simulink model "cllc_control"  (R2022a)
settings: Solver=FixedStepDiscrete  StartTime=0.0  StopTime=Inf  FixedStep=stepsize  RelTol=1e-9  AbsTol=1e-9  EnableMultiTasking=on
model workspace (MAT data in the model file):
  A_d = [1  1  1  1  1  1  1  1  1; 2  2  2  2  2  2  2  2  2]
  dcdc_direction = 1
  iout_ref = Simulink.Parameter
  iout_ref.DataType = 'auto'
  iout_ref.Complexity = 'real'
  iout_ref.Dimensions = [0 0]
  llc1_pri_idc = Simulink.Signal
  llc1_pri_idc.DataType = 'uint16'
  llc1_pri_idc.Dimensions = -1
  llc1_pri_idc.DimensionsMode = 'Fixed'
  llc1_pri_idc.Complexity = 'real'
  llc1_pri_idc.SampleTime = -1
  llc1_pri_idc.SamplingMode = 'auto'
  llc1_pri_idc.InitialValue = '0'
  llc1_sec_idc = Simulink.Signal
  llc1_sec_idc.DataType = 'uint16'
  llc1_sec_idc.Dimensions = -1
  llc1_sec_idc.DimensionsMode = 'Fixed'
  llc1_sec_idc.Complexity = 'real'
  llc1_sec_idc.SampleTime = -1
  llc1_sec_idc.SamplingMode = 'auto'
  llc1_sec_idc.InitialValue = '0'
  ref_iout = Simulink.Signal
  ref_iout.DataType = 'uint16'
  ref_iout.Dimensions = -1
  ref_iout.DimensionsMode = 'Fixed'
  ref_iout.Complexity = 'real'
  ref_iout.SampleTime = -1
  ref_iout.SamplingMode = 'auto'
  ref_iout.InitialValue = '0'
  ref_iout_calib = Simulink.Signal
  ref_iout_calib.DataType = 'uint16'
  ref_iout_calib.Dimensions = -1
  ref_iout_calib.DimensionsMode = 'Fixed'
  ref_iout_calib.Complexity = 'real'
  ref_iout_calib.SampleTime = -1
  ref_iout_calib.SamplingMode = 'auto'
  ref_iout_calib.InitialValue = '0'
  ref_ss_llc1 = Simulink.Signal
  ref_ss_llc1.DataType = 'uint16'
  ref_ss_llc1.Dimensions = -1
  ref_ss_llc1.DimensionsMode = 'Fixed'
  ref_ss_llc1.Complexity = 'real'
  ref_ss_llc1.SampleTime = -1
  ref_ss_llc1.SamplingMode = 'auto'
  ref_ss_llc1.InitialValue = '0'
  ref_vbat = Simulink.Signal
  ref_vbat.DataType = 'uint16'
  ref_vbat.Dimensions = -1
  ref_vbat.DimensionsMode = 'Fixed'
  ref_vbat.Complexity = 'real'
  ref_vbat.SampleTime = -1
  ref_vbat.SamplingMode = 'auto'
  ref_vbat.InitialValue = '0'
  ref_vbat_calib = Simulink.Signal
  ref_vbat_calib.DataType = 'uint16'
  ref_vbat_calib.Dimensions = -1
  ref_vbat_calib.DimensionsMode = 'Fixed'
  ref_vbat_calib.Complexity = 'real'
  ref_vbat_calib.SampleTime = -1
  ref_vbat_calib.SamplingMode = 'auto'
  ref_vbat_calib.InitialValue = '0'
  vbat = Simulink.Signal
  vbat.DataType = 'uint16'
  vbat.Dimensions = -1
  vbat.DimensionsMode = 'Fixed'
  vbat.Complexity = 'real'
  vbat.SampleTime = -1
  vbat.SamplingMode = 'auto'
  vbat.InitialValue = '0'
  vbat_ref = Simulink.Parameter
  vbat_ref.DataType = 'auto'
  vbat_ref.Complexity = 'real'
  vbat_ref.Dimensions = [0 0]
  vout = Simulink.Signal
  vout.DataType = 'uint16'
  vout.Dimensions = -1
  vout.DimensionsMode = 'Fixed'
  vout.Complexity = 'real'
  vout.SampleTime = -1
  vout.SamplingMode = 'auto'
  vout.InitialValue = '0'
values from neighbouring files (symbols this model uses):
  epwmclk = 100000000.0    [cllc_data_lib.sldd]
  stepsize = 2.0E-7    [cllc_data_lib.sldd]
  var_dir_v2g = 0.0    [cllc_data_lib.sldd]
undefined symbols (not defined in the file or in its folder): f32Iout, f32VoutTarget
libraries: spsSampleandHoldLib x16, simulink_extras x6
(part 1 of 2)
settings Model: DataDictionary=cllc_data_lib.sldd  EnableAccessToBaseWorkspace=off  ExtModeTrigDuration=8  Creator=johncanas  LastModifiedBy=sgcesuser2
settings SolverCC: MaxConsecutiveMinStep=10  ZeroCrossAlgorithm=Adaptive  AlgebraicLoopSolver=TrustRegion  AutoInsertRateTranBlk=on  InsertRTBMode=Always
settings DataIOCC: SaveState=on  SignalLoggingName=SIL_signals
settings OptimizationCC: DefaultUnderspecifiedDataType=single  EnhancedBackFolding=on  PassReuseOutputArgsAs=Individual arguments  MaxStackSize=1024  OptimizeBlockOrder=speed  DifferentSizesBufferReuse=on  OptimizationCustomize=off  DenormalBehavior=FlushToZero  EfficientTunableParamExpr=on
settings DebuggingCC: IgnoredZcDiagnostic=none  MultiTaskDSMMsg=none  ParameterTunabilityLossMsg=error  UnconnectedInputMsg=warning  UnconnectedOutputMsg=warning  UnconnectedLineMsg=warning  BusObjectLabelMismatch=error  SFMachineParentedDataDiag=warning  UnderSpecifiedDimensionMsg=warning
settings HardwareCC: ProdBitPerChar=16  ProdBitPerInt=16  ProdBitPerPointer=32  ProdBitPerSizeT=32  ProdBitPerPtrDiffT=32  ProdLargestAtomicInteger=Integer  ProdLargestAtomicFloat=None  ProdWordSize=16  ProdLongLongMode=on  ProdHWDeviceType=Texas Instruments->C2000
settings ModelReferenceCC: EnableRefExpFcnMdlSchedulingChecks=off
settings SFSimCC: MATLABDynamicMemAlloc=off  CustomCodeUndefinedFunction=UseInterfaceOnly
settings RTWCC: SystemTargetFile=ert.tlc  HardwareBoard=TI Piccolo F2807x  TemplateMakefile=ert_default_tmf  GenerateReport=on  Toolchain=Texas Instruments Code Composer Studio (C2000)  IncludeHyperlinkInReport=on  LaunchReport=on  PortableWordSizes=on  GenerateTraceInfo=on  GenerateTraceReport=on  GenerateTraceReportSl=on  GenerateTraceReportSf=on  GenerateTraceReportEml=on  DLArmComputeVersion=19.05
settings CodeAppCC: ForceParamTrailComments=on  IgnoreCustomStorageClasses=off  OperatorAnnotations=on  SimulinkDataObjDesc=on  SFDataObjDesc=on  InsertBlockDesc=on
settings ERTTargetCC: CodeReplacementLibrary=TI C28x  SupportContinuousTime=on  SupportNonInlinedSFcns=on  ExtModeStaticAllocSize=2000

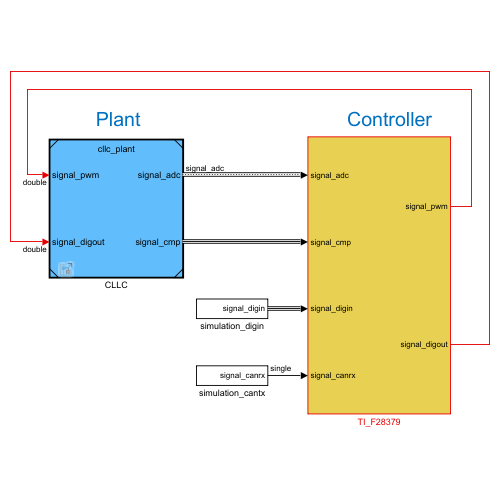
[thumbnail: Simulink's stored preview of the top-level diagram]
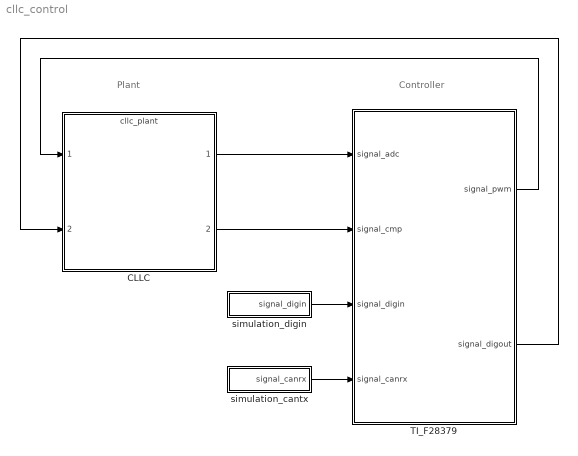
== system cllc_control ==
  note: Controller
  note: Plant
  CLLC : ModelReference  ModelNameDialog=cllc_plant.slx  SimulationMode=Normal  ModelReferenceVersion=2.76
  TI_F28379 : Subsystem
  simulation_cantx : Subsystem
  simulation_digin : Subsystem
  wires:
  CLLC/1 -> TI_F28379/1(signal_adc)
  TI_F28379/1(signal_pwm) -> CLLC/1
  TI_F28379/2(signal_digout) -> CLLC/2
  CLLC/2 -> TI_F28379/2(signal_cmp)
  simulation_digin/1(signal_digin) -> TI_F28379/3(signal_digin)
  simulation_cantx/1(signal_canrx) -> TI_F28379/4(signal_canrx)

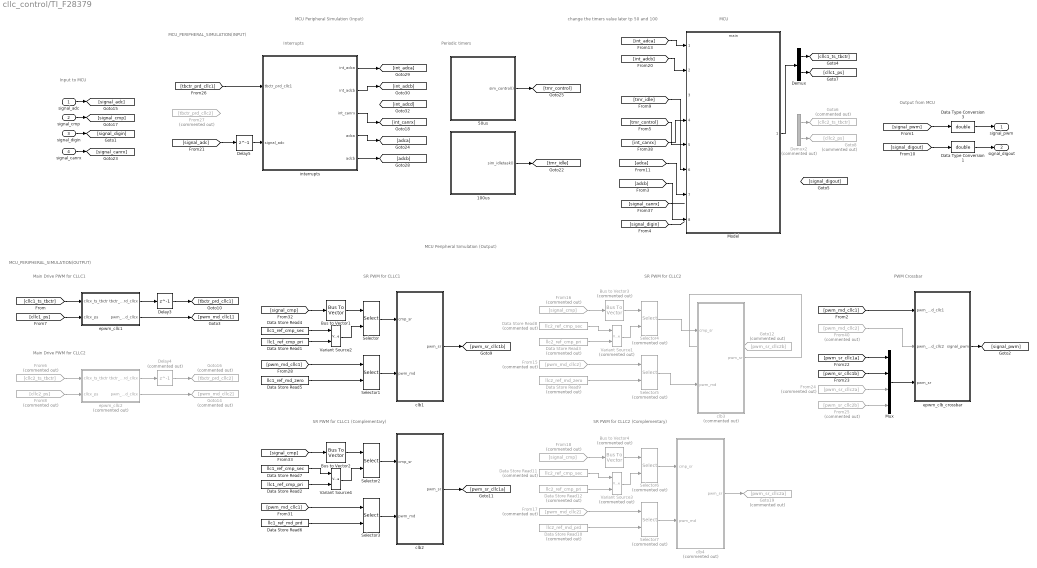
== system cllc_control/TI_F28379 ==
  note: change the timers value later tp 50 and 100
  note: MCU_PERIPHERAL_SIMULATION(OUTPUT)
  note: MCU_PERIPHERAL_SIMULATION(INPUT)
  note: MCU
  note: Input to MCU
  note: Output from MCU
  note: Interrupts
  note: Periodic timers
  note: SR PWM for CLLC2 (Complementary)
  note: SR PWM for CLLC2
  note: Main Drive PWM for CLLC2
  note: SR PWM for CLLC1 (Complementary)
  note: SR PWM for CLLC1
  note: Main Drive PWM for CLLC1
  note: PWM Crossbar
  note: MCU Peripheral Simulation (Input)
  note: MCU Peripheral Simulation (Output)
  signal_adc : Inport
  signal_cmp : Inport  Port=2
  signal_digin : Inport  Port=3
  signal_canrx : Inport  Port=4
  100us : Stateflow chart  TreatAsAtomicUnit=on  SystemSampleTime=2e-6
  50us : Stateflow chart  TreatAsAtomicUnit=on  SystemSampleTime=50e-6
  Bus to Vector1 : BusToVector
  Bus to Vector2 : BusToVector
  Bus to Vector3 : BusToVector  Commented=on
  Bus to Vector4 : BusToVector  Commented=on
  Data Store Read1 : DataStoreRead  DataStoreName=llc1_ref_cmp_pri  IndexOptions=Index vector (dialog)  Indices=1  OutputSizes=1
  Data Store Read10 : DataStoreRead  Commented=on  DataStoreName=llc2_ref_md_prd  IndexOptions=Index vector (dialog)  Indices=1  OutputSizes=1
  Data Store Read11 : DataStoreRead  Commented=on  DataStoreName=llc2_ref_cmp_sec  IndexOptions=Index vector (dialog)  Indices=1  OutputSizes=1
  Data Store Read12 : DataStoreRead  Commented=on  DataStoreName=llc2_ref_cmp_pri  IndexOptions=Index vector (dialog)  Indices=1  OutputSizes=1
  Data Store Read2 : DataStoreRead  DataStoreName=llc1_ref_cmp_pri  IndexOptions=Index vector (dialog)  Indices=1  OutputSizes=1
  Data Store Read3 : DataStoreRead  Commented=on  DataStoreName=llc2_ref_cmp_pri  IndexOptions=Index vector (dialog)  Indices=1  OutputSizes=1
  Data Store Read4 : DataStoreRead  DataStoreName=llc1_ref_cmp_sec  IndexOptions=Index vector (dialog)  Indices=1  OutputSizes=1
  Data Store Read5 : DataStoreRead  DataStoreName=llc1_ref_md_zero  IndexOptions=Index vector (dialog)  Indices=1  OutputSizes=1
  Data Store Read6 : DataStoreRead  DataStoreName=llc1_ref_md_prd  IndexOptions=Index vector (dialog)  Indices=1  OutputSizes=1
  Data Store Read7 : DataStoreRead  DataStoreName=llc1_ref_cmp_sec  IndexOptions=Index vector (dialog)  Indices=1  OutputSizes=1
  Data Store Read8 : DataStoreRead  Commented=on  DataStoreName=llc2_ref_cmp_sec  IndexOptions=Index vector (dialog)  Indices=1  OutputSizes=1
  Data Store Read9 : DataStoreRead  Commented=on  DataStoreName=llc2_ref_md_zero  IndexOptions=Index vector (dialog)  Indices=1  OutputSizes=1
  Data Type Conversion1 : DataTypeConversion  OutDataTypeStr=double  SaturateOnIntegerOverflow=off  RndMeth=Floor
  Data Type Conversion3 : DataTypeConversion  OutDataTypeStr=double  SaturateOnIntegerOverflow=off  RndMeth=Floor
  Delay3 : Delay  DelayLength=1
  Delay4 : Delay  Commented=on  DelayLength=1
  Delay5 : Delay  DelayLength=1
  Demux : Demux  Outputs=2
  Demux2 : Demux  Commented=on  Outputs=2
  From15 : From  Commented=on  GotoTag=pwm_md_cllc2
  From16 : From  Commented=on  GotoTag=signal_cmp
  From17 : From  Commented=on  GotoTag=pwm_md_cllc2
  From18 : From  Commented=on  GotoTag=signal_cmp
  From24 : From  Commented=on  GotoTag=pwm_sr_cllc2a
  From25 : From  Commented=on  GotoTag=pwm_sr_cllc2b
  From27 : From  Commented=on  GotoTag=tbctr_prd_cllc2
  From40 : From  Commented=on  GotoTag=pwm_md_cllc2
  From6 : From  Commented=on  GotoTag=cllc2_ts_tbctr
  From8 : From  Commented=on  GotoTag=cllc2_ps
  Goto12 : Goto  Commented=on  GotoTag=pwm_sr_cllc2b
  Goto14 : Goto  Commented=on  GotoTag=pwm_md_cllc2
  Goto16 : Goto  Commented=on  GotoTag=tbctr_prd_cllc2
  Goto19 : Goto  Commented=on  GotoTag=pwm_sr_cllc2a
  Goto6 : Goto  Commented=on  GotoTag=cllc2_ts_tbctr
  Goto8 : Goto  Commented=on  GotoTag=cllc2_ps
  Model : ModelReference  ModelNameDialog=main.slx  SimulationMode=Normal  ScheduleRates=on  ModelReferenceVersion=5.515
  Mux : Mux
  Selector : Selector  InputPortWidth=4  IndexOptions=Index vector (port)  Indices=[1 3]  OutputSizes=1
  Selector1 : Selector  InputPortWidth=8  IndexOptions=Index vector (port)  Indices=[1 3]  OutputSizes=1
  Selector2 : Selector  InputPortWidth=4  IndexOptions=Index vector (port)  Indices=[1 3]  OutputSizes=1
  Selector3 : Selector  InputPortWidth=8  IndexOptions=Index vector (port)  Indices=[1 3]  OutputSizes=1
  Selector4 : Selector  Commented=on  InputPortWidth=4  IndexOptions=Index vector (port)  Indices=[1 3]  OutputSizes=1
  Selector5 : Selector  Commented=on  InputPortWidth=8  IndexOptions=Index vector (port)  Indices=[1 3]  OutputSizes=1
  Selector6 : Selector  Commented=on  InputPortWidth=4  IndexOptions=Index vector (port)  Indices=[1 3]  OutputSizes=1
  Selector7 : Selector  Commented=on  InputPortWidth=8  IndexOptions=Index vector (port)  Indices=[1 3]  OutputSizes=1
  Variant Source1 : VariantSource  Commented=on
      settings: AllowZeroVariantControls=on
  Variant Source2 : VariantSource
      settings: AllowZeroVariantControls=on
  Variant Source3 : VariantSource  Commented=on
      settings: AllowZeroVariantControls=on
  Variant Source4 : VariantSource
      settings: AllowZeroVariantControls=on
  clb1 : Subsystem
  clb2 : Subsystem
  clb3 : Subsystem  Commented=on
  clb4 : Subsystem  Commented=on
  epwm_clb_crossbar : Subsystem
  epwm_cllc1 : Subsystem
  epwm_cllc2 : Subsystem  Commented=on
  interrupts : Subsystem
  signal_pwm : Outport  VectorParamsAs1DForOutWhenUnconnected=off
  signal_digout : Outport  Port=2
  wires:
  Model/1 -> Demux/1
  Demux/1 -> [cllc1_ts_tbctr]
  Demux/2 -> [cllc1_ps]
  [signal_digout] -> Data Type Conversion1/1
  Demux2/2 -> Goto8/1
  Demux2/1 -> Goto6/1
  signal_cmp/1 -> [signal_cmp]
  ? -> [signal_digout]
  signal_adc/1 -> [signal_adc]
  [int_adca] -> Model/1
  [int_adcb] -> Model/2
  ? -> Model/3
  signal_digin/1 -> [signal_digin]
  signal_canrx/1 -> [signal_canrx]
  [signal_digin] -> ?
  [signal_canrx] -> ?
  ? -> [int_adcd]
  interrupts/5(adcb) -> [adcb]
  interrupts/4(adca) -> [adca]
  Delay5/1 -> interrupts/2(signal_adc)
  [tbctr_prd_cllc1] -> interrupts/1(tbctr_prd_cllc1)
  interrupts/3(int_canrx) -> [int_canrx]
  interrupts/1(int_adca) -> [int_adca]
  50us/1(sim_control()) -> [tmr_control]
  [signal_adc] -> Delay5/1
  interrupts/2(int_adcb) -> [int_adcb]
  100us/1(sim_idletask()) -> [tmr_idle]
  [signal_pwm] -> Data Type Conversion3/1
  Data Type Conversion3/1 -> signal_pwm/1
  Selector4/1 -> clb3/1(cmp_sr)
  From16/1 -> Bus to Vector3/1
  Selector6/1 -> clb4/1(cmp_sr)
  Bus to Vector3/1 -> Selector4/1
  [pwm_md_cllc1] -> Selector1/1
  From18/1 -> Bus to Vector4/1
  Delay3/1 -> [tbctr_prd_cllc1]
  Bus to Vector1/1 -> Selector/1
  Data Store Read7/1 -> Variant Source4/1
  From24/1 -> Mux/3
  Selector3/1 -> clb2/2(pwm_md)
  Bus to Vector4/1 -> Selector6/1
  Delay4/1 -> Goto16/1
  Bus to Vector2/1 -> Selector2/1
  From25/1 -> Mux/4
  Selector7/1 -> clb4/2(pwm_md)
  Selector1/1 -> clb1/2(pwm_md)
  clb4/1(pwm_sr) -> Goto19/1
  epwm_clb_crossbar/1(signal_pwm) -> [signal_pwm]
  From15/1 -> Selector5/1
  epwm_cllc1/1(tbctr_prd_cllcx) -> Delay3/1
  Data Store Read8/1 -> Variant Source1/1
  epwm_cllc2/1(tbctr_prd_cllcx) -> Delay4/1
  [pwm_md_cllc1] -> Selector3/1
  Selector5/1 -> clb3/2(pwm_md)
  clb2/1(pwm_sr) -> [pwm_sr_cllc1a]
  epwm_cllc2/2(pwm_md_cllcx) -> Goto14/1
  [pwm_sr_cllc1a] -> Mux/1
  From8/1 -> epwm_cllc2/2(cllcx_ps)
  From6/1 -> epwm_cllc2/1(cllcx_ts_tbctr)
  [signal_cmp] -> Bus to Vector2/1
  Data Store Read10/1 -> Selector7/2
  Selector2/1 -> clb2/1(cmp_sr)
  Data Store Read11/1 -> Variant Source3/1
  [signal_cmp] -> Bus to Vector1/1
  Mux/1 -> epwm_clb_crossbar/3(pwm_sr)
  clb3/1(pwm_sr) -> Goto12/1
  [cllc1_ps] -> epwm_cllc1/2(cllcx_ps)
  [pwm_sr_cllc1b] -> Mux/2
  clb1/1(pwm_sr) -> [pwm_sr_cllc1b]
  [pwm_md_cllc1] -> epwm_clb_crossbar/1(pwm_md_cllc1)
  epwm_cllc1/2(pwm_md_cllcx) -> [pwm_md_cllc1]
  Selector/1 -> clb1/1(cmp_sr)
  From17/1 -> Selector7/1
  Data Store Read4/1 -> Variant Source2/1
  [cllc1_ts_tbctr] -> epwm_cllc1/1(cllcx_ts_tbctr)
  Data Store Read9/1 -> Selector5/2
  From40/1 -> epwm_clb_crossbar/2(pwm_md_cllc2)
  Variant Source2/1 -> Selector/2
  Data Store Read1/1 -> Variant Source2/2
  Variant Source3/1 -> Selector6/2
  Variant Source1/1 -> Selector4/2
  Variant Source4/1 -> Selector2/2
  Data Store Read2/1 -> Variant Source4/2
  Data Store Read3/1 -> Variant Source1/2
  Data Store Read12/1 -> Variant Source3/2
  Data Type Conversion1/1 -> signal_digout/1
  Data Store Read5/1 -> Selector1/2
  Data Store Read6/1 -> Selector3/2
  [int_canrx] -> Model/4
  [tmr_idle] -> Model/6
  [tmr_control] -> Model/5
  [adca] -> Model/7
  [adcb] -> Model/8

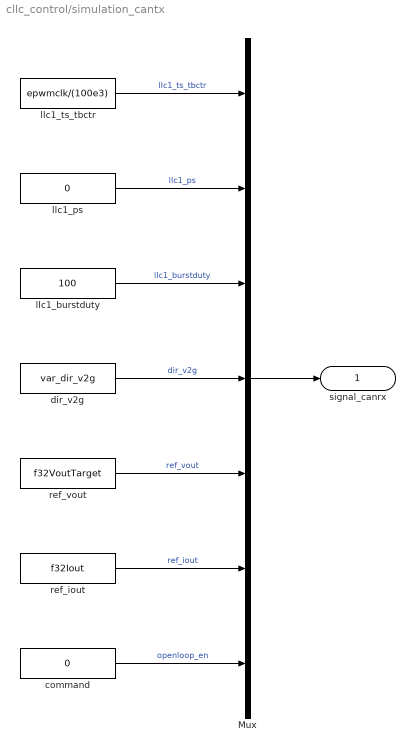
== system cllc_control/simulation_cantx ==
  Mux : Mux  Inputs=7
  command : Constant  Value=0  OutDataTypeStr=single
  dir_v2g : Constant  Value=var_dir_v2g  OutDataTypeStr=single
  llc1_burstduty : Constant  Value=100  OutDataTypeStr=single
  llc1_ps : Constant  Value=0  OutDataTypeStr=single
  llc1_ts_tbctr : Constant  Value=epwmclk/(100e3)  OutDataTypeStr=single
  ref_iout : Constant  Value=f32Iout  OutDataTypeStr=single
  ref_vout : Constant  Value=f32VoutTarget  OutDataTypeStr=single
  signal_canrx : Outport  VectorParamsAs1DForOutWhenUnconnected=off
  wires:
  ref_iout/1 -> Mux/6  "ref_iout"
  ref_vout/1 -> Mux/5  "ref_vout"
  Mux/1 -> signal_canrx/1
  dir_v2g/1 -> Mux/4  "dir_v2g"
  command/1 -> Mux/7  "openloop_en"
  llc1_ps/1 -> Mux/2  "llc1_ps"
  llc1_burstduty/1 -> Mux/3  "llc1_burstduty"
  llc1_ts_tbctr/1 -> Mux/1  "llc1_ts_tbctr"

== system cllc_control/simulation_digin ==
  Bus Creator : BusCreator  Inputs=7  OutDataTypeStr=Bus: signal_digin
  ac_ok : Constant  OutDataTypeStr=boolean
  can_addr{1..4} (4 alike) : Constant  Value=0  OutDataTypeStr=boolean
  dcdc_en : Constant  OutDataTypeStr=boolean
  pfc_ok : Constant  OutDataTypeStr=boolean
  signal_digin : Outport  VectorParamsAs1DForOutWhenUnconnected=off
  wires:
  Bus Creator/1 -> signal_digin/1
  can_addr1/1 -> Bus Creator/1  "can_addr1"
  can_addr2/1 -> Bus Creator/2  "can_addr2"
  dcdc_en/1 -> Bus Creator/7  "dcdc_en"
  ac_ok/1 -> Bus Creator/6  "ac_ok"
  pfc_ok/1 -> Bus Creator/5  "pfc_ok"
  can_addr4/1 -> Bus Creator/4  "can_addr4"
  can_addr3/1 -> Bus Creator/3  "can_addr3"

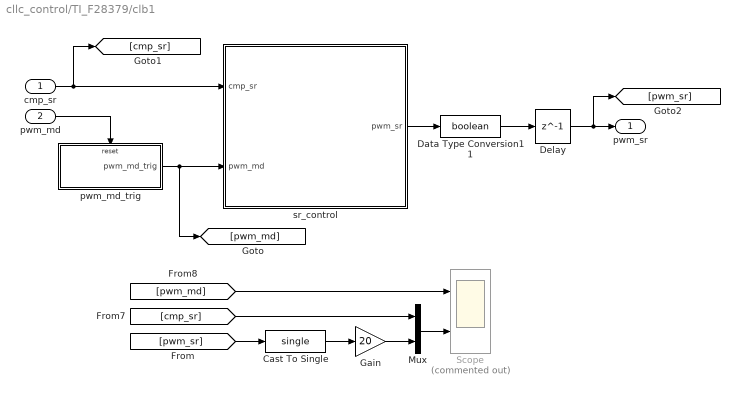
== system cllc_control/TI_F28379/clb1 ==
  cmp_sr : Inport
  pwm_md : Inport  Port=2
  Cast To Single : DataTypeConversion  OutDataTypeStr=single  SaturateOnIntegerOverflow=off  RndMeth=Floor
  Data Type Conversion11 : DataTypeConversion  OutDataTypeStr=boolean  SaturateOnIntegerOverflow=off  RndMeth=Floor
  Delay : Delay  DelayLength=1
  Gain : Gain  Gain=20
  Mux : Mux  Inputs=2
  Scope : Scope  Commented=on  NumInputPorts=2
  pwm_md_trig : Subsystem  TreatAsAtomicUnit=on
  sr_control : Stateflow chart  TreatAsAtomicUnit=on
  pwm_sr : Outport
  wires:
  [pwm_md] -> Scope/1
  [cmp_sr] -> Mux/1
  pwm_md_trig/1(pwm_md_trig) -> sr_control/2(pwm_md), [pwm_md]
  cmp_sr/1 -> sr_control/1(cmp_sr), [cmp_sr]
  Data Type Conversion11/1 -> Delay/1
  Delay/1 -> [pwm_sr], pwm_sr/1
  sr_control/1(pwm_sr) -> Data Type Conversion11/1
  pwm_md/1 -> pwm_md_trig/Reset
  Mux/1 -> Scope/2
  [pwm_sr] -> Cast To Single/1
  Cast To Single/1 -> Gain/1
  Gain/1 -> Mux/2

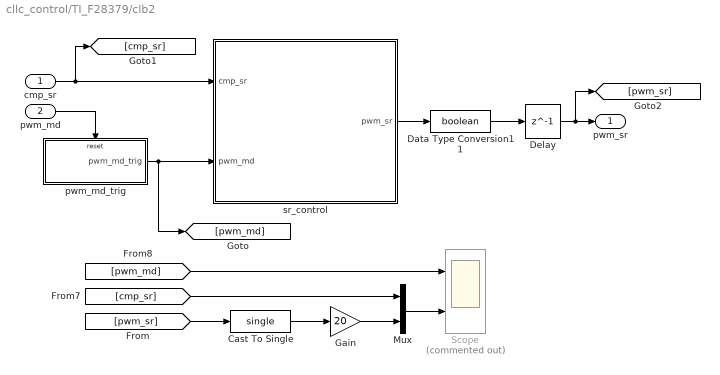
== system cllc_control/TI_F28379/clb2 ==
  cmp_sr : Inport
  pwm_md : Inport  Port=2
  Cast To Single : DataTypeConversion  OutDataTypeStr=single  SaturateOnIntegerOverflow=off  RndMeth=Floor
  Data Type Conversion11 : DataTypeConversion  OutDataTypeStr=boolean  SaturateOnIntegerOverflow=off  RndMeth=Floor
  Delay : Delay  DelayLength=1
  Gain : Gain  Gain=20
  Mux : Mux  Inputs=2
  Scope : Scope  Commented=on  NumInputPorts=2
  pwm_md_trig : Subsystem  TreatAsAtomicUnit=on
  sr_control : Stateflow chart  TreatAsAtomicUnit=on
  pwm_sr : Outport
  wires:
  Gain/1 -> Mux/2
  Cast To Single/1 -> Gain/1
  [pwm_sr] -> Cast To Single/1
  Mux/1 -> Scope/2
  pwm_md/1 -> pwm_md_trig/Reset
  sr_control/1(pwm_sr) -> Data Type Conversion11/1
  Delay/1 -> pwm_sr/1, [pwm_sr]
  Data Type Conversion11/1 -> Delay/1
  cmp_sr/1 -> sr_control/1(cmp_sr), [cmp_sr]
  pwm_md_trig/1(pwm_md_trig) -> sr_control/2(pwm_md), [pwm_md]
  [cmp_sr] -> Mux/1
  [pwm_md] -> Scope/1

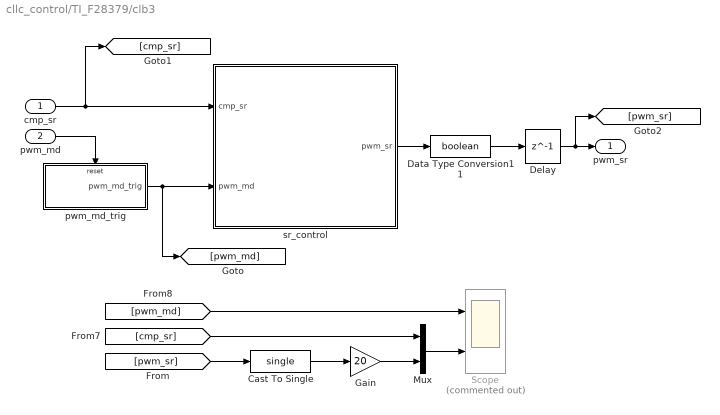
== system cllc_control/TI_F28379/clb3 ==
  cmp_sr : Inport
  pwm_md : Inport  Port=2
  Cast To Single : DataTypeConversion  OutDataTypeStr=single  SaturateOnIntegerOverflow=off  RndMeth=Floor
  Data Type Conversion11 : DataTypeConversion  OutDataTypeStr=boolean  SaturateOnIntegerOverflow=off  RndMeth=Floor
  Delay : Delay  DelayLength=1
  Gain : Gain  Gain=20
  Mux : Mux  Inputs=2
  Scope : Scope  Commented=on  NumInputPorts=2
  pwm_md_trig : Subsystem  TreatAsAtomicUnit=on
  sr_control : Stateflow chart  TreatAsAtomicUnit=on
  pwm_sr : Outport
  wires:
  Gain/1 -> Mux/2
  Cast To Single/1 -> Gain/1
  [pwm_sr] -> Cast To Single/1
  Mux/1 -> Scope/2
  pwm_md/1 -> pwm_md_trig/Reset
  sr_control/1(pwm_sr) -> Data Type Conversion11/1
  Delay/1 -> pwm_sr/1, [pwm_sr]
  Data Type Conversion11/1 -> Delay/1
  cmp_sr/1 -> sr_control/1(cmp_sr), [cmp_sr]
  pwm_md_trig/1(pwm_md_trig) -> sr_control/2(pwm_md), [pwm_md]
  [cmp_sr] -> Mux/1
  [pwm_md] -> Scope/1

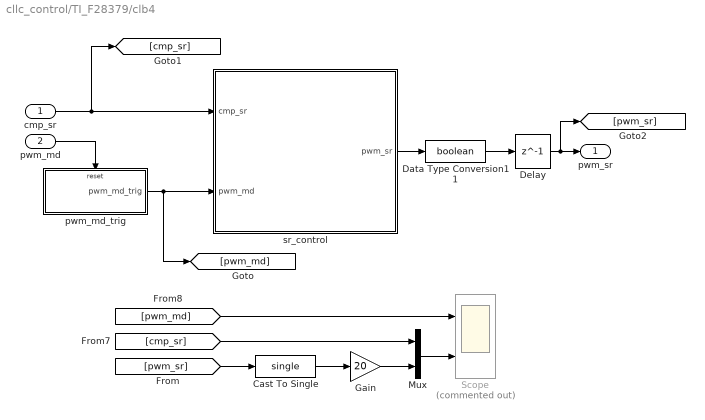
== system cllc_control/TI_F28379/clb4 ==
  cmp_sr : Inport
  pwm_md : Inport  Port=2
  Cast To Single : DataTypeConversion  OutDataTypeStr=single  SaturateOnIntegerOverflow=off  RndMeth=Floor
  Data Type Conversion11 : DataTypeConversion  OutDataTypeStr=boolean  SaturateOnIntegerOverflow=off  RndMeth=Floor
  Delay : Delay  DelayLength=1
  Gain : Gain  Gain=20
  Mux : Mux  Inputs=2
  Scope : Scope  Commented=on  NumInputPorts=2
  pwm_md_trig : Subsystem  TreatAsAtomicUnit=on
  sr_control : Stateflow chart  TreatAsAtomicUnit=on
  pwm_sr : Outport
  wires:
  [pwm_md] -> Scope/1
  [cmp_sr] -> Mux/1
  pwm_md_trig/1(pwm_md_trig) -> sr_control/2(pwm_md), [pwm_md]
  cmp_sr/1 -> sr_control/1(cmp_sr), [cmp_sr]
  Data Type Conversion11/1 -> Delay/1
  Delay/1 -> [pwm_sr], pwm_sr/1
  sr_control/1(pwm_sr) -> Data Type Conversion11/1
  pwm_md/1 -> pwm_md_trig/Reset
  Mux/1 -> Scope/2
  [pwm_sr] -> Cast To Single/1
  Cast To Single/1 -> Gain/1
  Gain/1 -> Mux/2

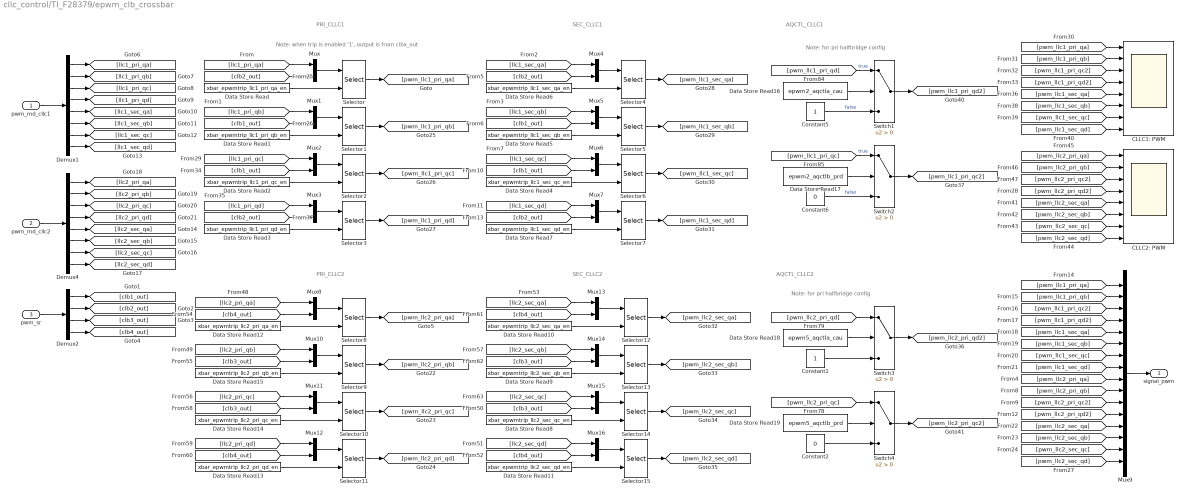
== system cllc_control/TI_F28379/epwm_clb_crossbar ==
  note: Note: when trip is enabled '1', output is from clbx_out
  note: PRI_CLLC1
  note: SEC_CLLC1
  note: PRI_CLLC2
  note: SEC_CLLC2
  note: Note: for pri halfbridge config
  note: AQCTL_CLLC2
  note: Note: for pri halfbridge config
  note: AQCTL_CLLC1
  pwm_md_cllc1 : Inport
  pwm_md_cllc2 : Inport  Port=2
  pwm_sr : Inport  Port=3
  CLLC1: PWM : Scope  NumInputPorts=8
  CLLC2: PWM : Scope  NumInputPorts=8
  Constant1 : Constant  OutDataTypeStr=boolean
  Constant2 : Constant  Value=0  OutDataTypeStr=boolean
  Constant5 : Constant  OutDataTypeStr=boolean
  Constant6 : Constant  Value=0  OutDataTypeStr=boolean
  Data Store Read : DataStoreRead  DataStoreName=xbar_epwmtrip_llc1_pri_qa_en  IndexOptions=Index vector (dialog)  Indices=1  OutputSizes=1
  Data Store Read1 : DataStoreRead  DataStoreName=xbar_epwmtrip_llc1_pri_qb_en  IndexOptions=Index vector (dialog)  Indices=1  OutputSizes=1
  Data Store Read10 : DataStoreRead  DataStoreName=xbar_epwmtrip_llc2_sec_qa_en  IndexOptions=Index vector (dialog)  Indices=1  OutputSizes=1
  Data Store Read11 : DataStoreRead  DataStoreName=xbar_epwmtrip_llc2_sec_qd_en  IndexOptions=Index vector (dialog)  Indices=1  OutputSizes=1
  Data Store Read12 : DataStoreRead  DataStoreName=xbar_epwmtrip_llc2_pri_qa_en  IndexOptions=Index vector (dialog)  Indices=1  OutputSizes=1
  Data Store Read13 : DataStoreRead  DataStoreName=xbar_epwmtrip_llc2_pri_qd_en  IndexOptions=Index vector (dialog)  Indices=1  OutputSizes=1
  Data Store Read14 : DataStoreRead  DataStoreName=xbar_epwmtrip_llc2_pri_qc_en  IndexOptions=Index vector (dialog)  Indices=1  OutputSizes=1
  Data Store Read15 : DataStoreRead  DataStoreName=xbar_epwmtrip_llc2_pri_qb_en  IndexOptions=Index vector (dialog)  Indices=1  OutputSizes=1
  Data Store Read16 : DataStoreRead  DataStoreName=epwm2_aqctla_cau  IndexOptions=Index vector (dialog)  Indices=1  OutputSizes=1
  Data Store Read17 : DataStoreRead  DataStoreName=epwm2_aqctlb_prd  IndexOptions=Index vector (dialog)  Indices=1  OutputSizes=1
  Data Store Read18 : DataStoreRead  DataStoreName=epwm5_aqctla_cau  IndexOptions=Index vector (dialog)  Indices=1  OutputSizes=1
  Data Store Read19 : DataStoreRead  DataStoreName=epwm5_aqctlb_prd  IndexOptions=Index vector (dialog)  Indices=1  OutputSizes=1
  Data Store Read2 : DataStoreRead  DataStoreName=xbar_epwmtrip_llc1_pri_qc_en  IndexOptions=Index vector (dialog)  Indices=1  OutputSizes=1
  Data Store Read3 : DataStoreRead  DataStoreName=xbar_epwmtrip_llc1_pri_qd_en  IndexOptions=Index vector (dialog)  Indices=1  OutputSizes=1
  Data Store Read4 : DataStoreRead  DataStoreName=xbar_epwmtrip_llc1_sec_qc_en  IndexOptions=Index vector (dialog)  Indices=1  OutputSizes=1
  Data Store Read5 : DataStoreRead  DataStoreName=xbar_epwmtrip_llc1_sec_qb_en  IndexOptions=Index vector (dialog)  Indices=1  OutputSizes=1
  Data Store Read6 : DataStoreRead  DataStoreName=xbar_epwmtrip_llc1_sec_qa_en  IndexOptions=Index vector (dialog)  Indices=1  OutputSizes=1
  Data Store Read7 : DataStoreRead  DataStoreName=xbar_epwmtrip_llc1_sec_qd_en  IndexOptions=Index vector (dialog)  Indices=1  OutputSizes=1
  Data Store Read8 : DataStoreRead  DataStoreName=xbar_epwmtrip_llc2_sec_qc_en  IndexOptions=Index vector (dialog)  Indices=1  OutputSizes=1
  Data Store Read9 : DataStoreRead  DataStoreName=xbar_epwmtrip_llc2_sec_qb_en  IndexOptions=Index vector (dialog)  Indices=1  OutputSizes=1
  Demux1 : Demux  Outputs=8
  Demux2 : Demux
  Demux4 : Demux  Outputs=8
  Mux{,1..8,10..16} (16 alike) : Mux  Inputs=2
  Mux9 : Mux  Inputs=16
  Selector{,1..15} (16 alike) : Selector  IndexMode=Zero-based  InputPortWidth=2  IndexOptions=Index vector (port)  Indices=[1 3]  OutputSizes=1
  Switch{1..4} (4 alike) : Switch  Criteria=u2 > Threshold  SaturateOnIntegerOverflow=off  InputSameDT=off
  signal_pwm : Outport
  wires:
  pwm_sr/1 -> Demux2/1
  pwm_md_cllc1/1 -> Demux1/1
  Demux1/1 -> [llc1_pri_qa]
  Demux1/2 -> [llc1_pri_qb]
  Demux1/8 -> [llc1_sec_qd]
  Demux1/7 -> [llc1_sec_qc]
  Demux1/6 -> [llc1_sec_qb]
  Demux1/5 -> [llc1_sec_qa]
  Demux1/4 -> [llc1_pri_qd]
  Demux1/3 -> [llc1_pri_qc]
  Demux4/3 -> [llc2_pri_qc]
  Demux4/4 -> [llc2_pri_qd]
  Demux4/5 -> [llc2_sec_qa]
  Demux4/6 -> [llc2_sec_qb]
  Demux4/7 -> [llc2_sec_qc]
  Demux4/8 -> [llc2_sec_qd]
  Demux4/2 -> [llc2_pri_qb]
  Demux4/1 -> [llc2_pri_qa]
  pwm_md_cllc2/1 -> Demux4/1
  Mux9/1 -> signal_pwm/1
  Data Store Read/1 -> Selector/2
  [clb2_out] -> Mux/2
  [llc1_pri_qa] -> Mux/1
  Mux/1 -> Selector/1
  Selector/1 -> [pwm_llc1_pri_qa]
  Mux1/1 -> Selector1/1
  [llc1_pri_qb] -> Mux1/1
  [clb1_out] -> Mux1/2
  Data Store Read1/1 -> Selector1/2
  Selector1/1 -> [pwm_llc1_pri_qb]
  Selector2/1 -> [pwm_llc1_pri_qc]
  Data Store Read2/1 -> Selector2/2
  [clb1_out] -> Mux2/2
  [llc1_pri_qc] -> Mux2/1
  Mux2/1 -> Selector2/1
  Mux3/1 -> Selector3/1
  [llc1_pri_qd] -> Mux3/1
  [clb2_out] -> Mux3/2
  Data Store Read3/1 -> Selector3/2
  Selector3/1 -> [pwm_llc1_pri_qd]
  Selector7/1 -> [pwm_llc1_sec_qd]
  Data Store Read7/1 -> Selector7/2
  [clb2_out] -> Mux7/2
  [llc1_sec_qd] -> Mux7/1
  Mux7/1 -> Selector7/1
  Mux6/1 -> Selector6/1
  [llc1_sec_qc] -> Mux6/1
  [clb1_out] -> Mux6/2
  Data Store Read4/1 -> Selector6/2
  Selector6/1 -> [pwm_llc1_sec_qc]
  Selector5/1 -> [pwm_llc1_sec_qb]
  Data Store Read5/1 -> Selector5/2
  [clb1_out] -> Mux5/2
  [llc1_sec_qb] -> Mux5/1
  Mux5/1 -> Selector5/1
  Selector4/1 -> [pwm_llc1_sec_qa]
  Mux4/1 -> Selector4/1
  [llc1_sec_qa] -> Mux4/1
  [clb2_out] -> Mux4/2
  Data Store Read6/1 -> Selector4/2
  [pwm_llc1_pri_qa] -> Mux9/1
  [pwm_llc1_pri_qb] -> Mux9/2
  [pwm_llc1_pri_qc2] -> Mux9/3
  [pwm_llc1_pri_qd2] -> Mux9/4
  [pwm_llc1_sec_qa] -> Mux9/5
  [pwm_llc1_sec_qb] -> Mux9/6
  [pwm_llc1_sec_qc] -> Mux9/7
  [pwm_llc1_sec_qd] -> Mux9/8
  Demux2/4 -> [clb4_out]
  Demux2/3 -> [clb3_out]
  Demux2/2 -> [clb2_out]
  Demux2/1 -> [clb1_out]
  [pwm_llc2_pri_qa] -> Mux9/9
  [pwm_llc2_pri_qb] -> Mux9/10
  [pwm_llc2_pri_qc2] -> Mux9/11
  [pwm_llc2_pri_qd2] -> Mux9/12
  [pwm_llc2_sec_qa] -> Mux9/13
  [pwm_llc2_sec_qb] -> Mux9/14
  [pwm_llc2_sec_qc] -> Mux9/15
  [pwm_llc2_sec_qd] -> Mux9/16
  [pwm_llc1_pri_qa] -> CLLC1: PWM/1
  [pwm_llc1_pri_qb] -> CLLC1: PWM/2
  [pwm_llc1_pri_qc2] -> CLLC1: PWM/3
  [pwm_llc1_pri_qd2] -> CLLC1: PWM/4
  [pwm_llc1_sec_qa] -> CLLC1: PWM/5
  [pwm_llc1_sec_qb] -> CLLC1: PWM/6
  [pwm_llc1_sec_qc] -> CLLC1: PWM/7
  [pwm_llc1_sec_qd] -> CLLC1: PWM/8
  [pwm_llc2_pri_qa] -> CLLC2: PWM/1
  [pwm_llc2_pri_qb] -> CLLC2: PWM/2
  [pwm_llc2_pri_qc2] -> CLLC2: PWM/3
  [pwm_llc2_pri_qd2] -> CLLC2: PWM/4
  [pwm_llc2_sec_qa] -> CLLC2: PWM/5
  [pwm_llc2_sec_qb] -> CLLC2: PWM/6
  [pwm_llc2_sec_qc] -> CLLC2: PWM/7
  [pwm_llc2_sec_qd] -> CLLC2: PWM/8
  Data Store Read10/1 -> Selector12/2
  [clb4_out] -> Mux13/2
  [llc2_sec_qa] -> Mux13/1
  Mux13/1 -> Selector12/1
  Selector12/1 -> [pwm_llc2_sec_qa]
  Mux14/1 -> Selector13/1
  [llc2_sec_qb] -> Mux14/1
  [clb3_out] -> Mux14/2
  Data Store Read9/1 -> Selector13/2
  Selector13/1 -> [pwm_llc2_sec_qb]
  Selector14/1 -> [pwm_llc2_sec_qc]
  Data Store Read8/1 -> Selector14/2
  [clb3_out] -> Mux15/2
  [llc2_sec_qc] -> Mux15/1
  Mux15/1 -> Selector14/1
  Mux16/1 -> Selector15/1
  [llc2_sec_qd] -> Mux16/1
  [clb4_out] -> Mux16/2
  Data Store Read11/1 -> Selector15/2
  Selector15/1 -> [pwm_llc2_sec_qd]
  Selector11/1 -> [pwm_llc2_pri_qd]
  Data Store Read13/1 -> Selector11/2
  [clb4_out] -> Mux12/2
  [llc2_pri_qd] -> Mux12/1
  Mux12/1 -> Selector11/1
  Mux11/1 -> Selector10/1
  [llc2_pri_qc] -> Mux11/1
  [clb3_out] -> Mux11/2
  Data Store Read14/1 -> Selector10/2
  Selector10/1 -> [pwm_llc2_pri_qc]
  Selector9/1 -> [pwm_llc2_pri_qb]
  Data Store Read15/1 -> Selector9/2
  [clb3_out] -> Mux10/2
  [llc2_pri_qb] -> Mux10/1
  Mux10/1 -> Selector9/1
  Selector8/1 -> [pwm_llc2_pri_qa]
  Mux8/1 -> Selector8/1
  [llc2_pri_qa] -> Mux8/1
  [clb4_out] -> Mux8/2
  Data Store Read12/1 -> Selector8/2
  [pwm_llc2_pri_qc] -> Switch4/1
  Constant2/1 -> Switch4/3
  [pwm_llc2_pri_qd] -> Switch3/1
  Constant1/1 -> Switch3/3
  Data Store Read18/1 -> Switch3/2
  Switch3/1 -> [pwm_llc2_pri_qd2]
  Data Store Read19/1 -> Switch4/2
  Data Store Read16/1 -> Switch1/2
  Constant5/1 -> Switch1/3  "false"
  [pwm_llc1_pri_qc] -> Switch2/1  "true"
  Constant6/1 -> Switch2/3  "false"
  Switch1/1 -> [pwm_llc1_pri_qd2]
  Data Store Read17/1 -> Switch2/2
  Switch4/1 -> [pwm_llc2_pri_qc2]
  [pwm_llc1_pri_qd] -> Switch1/1  "true"
  Switch2/1 -> [pwm_llc1_pri_qc2]

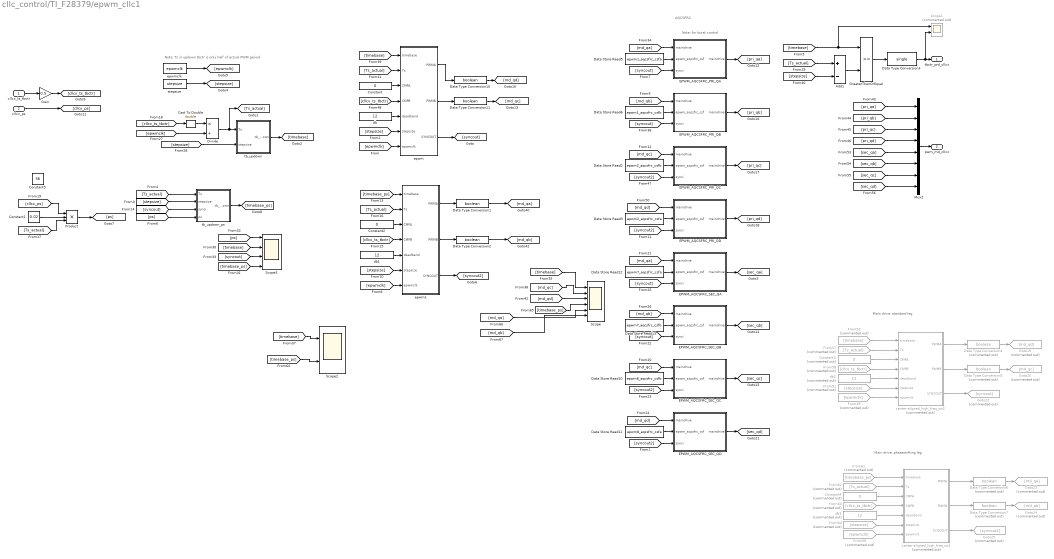
== system cllc_control/TI_F28379/epwm_cllc1 ==
  note: Note: Ts in updown tbctr is only half of actual PWM period
  note: Main drive: standard leg
  note: Main drive: phaseshifting leg
  note: AQCSFRC
  note: Note: for burst control
  cllcx_ts_tbctr : Inport
  cllcx_ps : Inport  Port=2
  Add1 : Sum  Inputs=+-
  Cast To Double : DataTypeConversion  OutDataTypeStr=double  SaturateOnIntegerOverflow=off  RndMeth=Floor
  Constant : Constant  Value=0
  Constant1 : Constant  Value=0.02
  Constant2 : Constant  Value=0
  Constant3 : Constant  Commented=on  Value=0
  Constant4 : Constant  Commented=on  Value=0
  Constant5 : Constant  Value=36
  Data Store Read10 : DataStoreRead  DataStoreName=epwm8_aqcsfrc_csfb  IndexOptions=Index vector (dialog)  Indices=1  OutputSizes=1
  Data Store Read11 : DataStoreRead  DataStoreName=epwm8_aqcsfrc_csfa  IndexOptions=Index vector (dialog)  Indices=1  OutputSizes=1
  Data Store Read12 : DataStoreRead  DataStoreName=epwm7_aqcsfrc_csfa  IndexOptions=Index vector (dialog)  Indices=1  OutputSizes=1
  Data Store Read13 : DataStoreRead  DataStoreName=epwm7_aqcsfrc_csfb  IndexOptions=Index vector (dialog)  Indices=1  OutputSizes=1
  Data Store Read2 : DataStoreRead  DataStoreName=epwm2_aqcsfrc_csfb  IndexOptions=Index vector (dialog)  Indices=1  OutputSizes=1
  Data Store Read3 : DataStoreRead  DataStoreName=epwm2_aqcsfrc_csfa  IndexOptions=Index vector (dialog)  Indices=1  OutputSizes=1
  Data Store Read5 : DataStoreRead  DataStoreName=epwm1_aqcsfrc_csfa  IndexOptions=Index vector (dialog)  Indices=1  OutputSizes=1
  Data Store Read6 : DataStoreRead  DataStoreName=epwm1_aqcsfrc_csfb  IndexOptions=Index vector (dialog)  Indices=1  OutputSizes=1
  Data Type Conversion{1..2,10..11} (4 alike) : DataTypeConversion  OutDataTypeStr=boolean  SaturateOnIntegerOverflow=off  RndMeth=Floor
  Data Type Conversion3 : DataTypeConversion  OutDataTypeStr=single  SaturateOnIntegerOverflow=off  RndMeth=Floor
  Data Type Conversion{4..7} (4 alike) : DataTypeConversion  Commented=on  OutDataTypeStr=boolean  SaturateOnIntegerOverflow=off  RndMeth=Floor
  Divide : Product  Inputs=*/
  EPWM_AQCSFRC_PRI_QA : Subsystem  TreatAsAtomicUnit=on
  EPWM_AQCSFRC_PRI_QB : Subsystem  TreatAsAtomicUnit=on
  EPWM_AQCSFRC_PRI_QC : Subsystem  TreatAsAtomicUnit=on
  EPWM_AQCSFRC_PRI_QD : Subsystem  TreatAsAtomicUnit=on
  EPWM_AQCSFRC_SEC_QA : Subsystem  TreatAsAtomicUnit=on
  EPWM_AQCSFRC_SEC_QB : Subsystem  TreatAsAtomicUnit=on
  EPWM_AQCSFRC_SEC_QC : Subsystem  TreatAsAtomicUnit=on
  EPWM_AQCSFRC_SEC_QD : Subsystem  TreatAsAtomicUnit=on
  From49 : From  Commented=on  GotoTag=epwmclk
  From51 : From  Commented=on  GotoTag=stepsize
  From52 : From  Commented=on  GotoTag=timebase
  From57 : From  Commented=on  GotoTag=Ts_actual
  From58 : From  Commented=on  GotoTag=cllcx_ts_tbctr
  From59 : From  Commented=on  GotoTag=epwmclk
  From60 : From  Commented=on  GotoTag=stepsize
  From61 : From  Commented=on  GotoTag=timebase_ps
  From62 : From  Commented=on  GotoTag=Ts_actual
  From63 : From  Commented=on  GotoTag=cllcx_ts_tbctr
  Gain : Gain  Gain=0.5
  Goto19 : Goto  Commented=on  GotoTag=md_qd
  Goto20 : Goto  Commented=on  GotoTag=md_qc
  Goto22 : Goto  Commented=on  GotoTag=syncout
  Goto23 : Goto  Commented=on  GotoTag=md_qa
  Goto24 : Goto  Commented=on  GotoTag=md_qb
  Goto25 : Goto  Commented=on  GotoTag=syncout2
  GreaterThanOrEqual : RelationalOperator  OutDataTypeStr=boolean  RndMeth=Simplest  InputSameDT=off
  Mux2 : Mux  Inputs=8
  Product : Product  Inputs=3  OutDataTypeStr=double
  Scope : Scope  NumInputPorts=6
  Scope1 : Scope  Commented=on  NumInputPorts=2
  Scope2 : Scope  NumInputPorts=2
  Scope3 : Scope  NumInputPorts=4
  center-aligned_high_freq_sw1 : MATLAB Function  Commented=on  TreatAsAtomicUnit=on
  center-aligned_high_freq_sw2 : MATLAB Function  Commented=on  TreatAsAtomicUnit=on
  db : Constant  Value=12
  db1 : Constant  Value=12
  db2 : Constant  Commented=on  Value=12
  db3 : Constant  Commented=on  Value=12
  epwm : MATLAB Function  TreatAsAtomicUnit=on
  epwm1 : MATLAB Function  TreatAsAtomicUnit=on
  epwmclk : Constant  Value=epwmclk
  stepsize : Constant  Value=stepsize
  tb_updown : Subsystem
  tb_updown_ps : Subsystem
  tbctr_prd_cllcx : Outport
  pwm_md_cllcx : Outport  Port=2
  wires:
  tb_updown/1(tb_updown) -> [timebase]
  Mux2/1 -> pwm_md_cllcx/1
  [cllcx_ts_tbctr] -> Cast To Double/1
  Divide/1 -> [Ts_actual], tb_updown/1(Ts)
  stepsize/1 -> [stepsize]
  [cllcx_ts_tbctr] -> epwm/4(CMPB)
  epwm/2(PWMB) -> Data Type Conversion11/1
  epwm/1(PWMA) -> Data Type Conversion10/1
  [Ts_actual] -> epwm/2(Ts)
  Constant/1 -> epwm/3(CMPA)
  [timebase] -> epwm/1(timebase)
  db/1 -> epwm/5(deadband)
  [stepsize] -> epwm/6(stepsize)
  epwmclk/1 -> [epwmclk]
  [epwmclk] -> epwm/7(epwmclk)
  cllcx_ps/1 -> [cllcx_ps]
  epwm/3(SYNCOUT) -> [syncout]
  tb_updown_ps/1(tb_updown) -> [timebase_ps]
  [stepsize] -> tb_updown_ps/2(stepsize)
  [Ts_actual] -> tb_updown_ps/1(Ts)
  [syncout] -> tb_updown_ps/3(synci)
  [ps] -> tb_updown_ps/4(ps)
  [epwmclk] -> epwm1/7(epwmclk)
  [stepsize] -> epwm1/6(stepsize)
  db1/1 -> epwm1/5(deadband)
  [timebase_ps] -> epwm1/1(timebase)
  Constant2/1 -> epwm1/3(CMPA)
  [Ts_actual] -> epwm1/2(Ts)
  epwm1/1(PWMA) -> Data Type Conversion1/1
  epwm1/2(PWMB) -> Data Type Conversion2/1
  [cllcx_ts_tbctr] -> epwm1/4(CMPB)
  [Ts_actual] -> Product/3
  Product/1 -> [ps]
  Constant1/1 -> Product/2
  cllcx_ts_tbctr/1 -> Gain/1
  [timebase] -> GreaterThanOrEqual/1, Scope1/1
  Data Type Conversion3/1 -> Scope1/2, tbctr_prd_cllcx/1
  GreaterThanOrEqual/1 -> Data Type Conversion3/1
  [epwmclk] -> Divide/2
  [stepsize] -> tb_updown/2(stepsize)
  [stepsize] -> Add1/2
  [Ts_actual] -> Add1/1
  Add1/1 -> GreaterThanOrEqual/2
  [timebase_ps] -> Scope3/4
  [syncout] -> Scope3/3
  [ps] -> Scope3/1
  [timebase] -> Scope3/2
  [syncout] -> EPWM_AQCSFRC_PRI_QA/3(synci)
  [md_qa] -> EPWM_AQCSFRC_PRI_QA/1(maindrive)
  [timebase] -> Scope/1
  [md_qc] -> Scope/2
  [md_qd] -> Scope/3
  Data Store Read5/1 -> EPWM_AQCSFRC_PRI_QA/2(epwm_aqcsfrc_csf)
  [md_qb] -> EPWM_AQCSFRC_PRI_QB/1(maindrive)
  Data Store Read6/1 -> EPWM_AQCSFRC_PRI_QB/2(epwm_aqcsfrc_csf)
  [syncout] -> EPWM_AQCSFRC_PRI_QB/3(synci)
  epwm1/3(SYNCOUT) -> [syncout2]
  [syncout2] -> EPWM_AQCSFRC_PRI_QD/3(synci)
  [syncout2] -> EPWM_AQCSFRC_PRI_QC/3(synci)
  Data Store Read2/1 -> EPWM_AQCSFRC_PRI_QC/2(epwm_aqcsfrc_csf)
  Data Store Read3/1 -> EPWM_AQCSFRC_PRI_QD/2(epwm_aqcsfrc_csf)
  [md_qd] -> EPWM_AQCSFRC_PRI_QD/1(maindrive)
  [md_qc] -> EPWM_AQCSFRC_PRI_QC/1(maindrive)
  EPWM_AQCSFRC_PRI_QA/1(maindrive') -> [pri_qa]
  EPWM_AQCSFRC_PRI_QB/1(maindrive') -> [pri_qb]
  EPWM_AQCSFRC_PRI_QC/1(maindrive') -> [pri_qc]
  EPWM_AQCSFRC_PRI_QD/1(maindrive') -> [pri_qd]
  [pri_qd] -> Mux2/4
  [pri_qc] -> Mux2/3
  [pri_qb] -> Mux2/2
  [pri_qa] -> Mux2/1
  [sec_qa] -> Mux2/5
  [sec_qb] -> Mux2/6
  [sec_qc] -> Mux2/7
  [sec_qd] -> Mux2/8
  EPWM_AQCSFRC_SEC_QD/1(maindrive') -> [sec_qd]
  EPWM_AQCSFRC_SEC_QC/1(maindrive') -> [sec_qc]
  EPWM_AQCSFRC_SEC_QB/1(maindrive') -> [sec_qb]
  EPWM_AQCSFRC_SEC_QA/1(maindrive') -> [sec_qa]
  [md_qc] -> EPWM_AQCSFRC_SEC_QC/1(maindrive)
  [md_qd] -> EPWM_AQCSFRC_SEC_QD/1(maindrive)
  Data Store Read11/1 -> EPWM_AQCSFRC_SEC_QD/2(epwm_aqcsfrc_csf)
  Data Store Read10/1 -> EPWM_AQCSFRC_SEC_QC/2(epwm_aqcsfrc_csf)
  [syncout2] -> EPWM_AQCSFRC_SEC_QC/3(synci)
  [syncout2] -> EPWM_AQCSFRC_SEC_QD/3(synci)
  [syncout] -> EPWM_AQCSFRC_SEC_QB/3(synci)
  Data Store Read13/1 -> EPWM_AQCSFRC_SEC_QB/2(epwm_aqcsfrc_csf)
  [md_qb] -> EPWM_AQCSFRC_SEC_QB/1(maindrive)
  Data Store Read12/1 -> EPWM_AQCSFRC_SEC_QA/2(epwm_aqcsfrc_csf)
  [md_qa] -> EPWM_AQCSFRC_SEC_QA/1(maindrive)
  [syncout] -> EPWM_AQCSFRC_SEC_QA/3(synci)
  Data Type Conversion1/1 -> [md_qa]
  Data Type Conversion2/1 -> [md_qb]
  Data Type Conversion10/1 -> [md_qd]
  Data Type Conversion11/1 -> [md_qc]
  Gain/1 -> [cllcx_ts_tbctr]
  db2/1 -> center-aligned_high_freq_sw2/5(deadband)
  Constant3/1 -> center-aligned_high_freq_sw2/3(CMPA)
  From57/1 -> center-aligned_high_freq_sw2/2(Ts)
  From49/1 -> center-aligned_high_freq_sw2/7(epwmclk)
  From58/1 -> center-aligned_high_freq_sw2/4(CMPB)
  From51/1 -> center-aligned_high_freq_sw2/6(stepsize)
  From52/1 -> center-aligned_high_freq_sw2/1(timebase)
  Data Type Conversion4/1 -> Goto19/1
  Data Type Conversion5/1 -> Goto20/1
  center-aligned_high_freq_sw2/1(PWMA) -> Data Type Conversion4/1
  center-aligned_high_freq_sw2/2(PWMB) -> Data Type Conversion5/1
  center-aligned_high_freq_sw2/3(SYNCOUT) -> Goto22/1
  center-aligned_high_freq_sw1/2(PWMB) -> Data Type Conversion7/1
  From60/1 -> center-aligned_high_freq_sw1/6(stepsize)
  Constant4/1 -> center-aligned_high_freq_sw1/3(CMPA)
  From61/1 -> center-aligned_high_freq_sw1/1(timebase)
  From59/1 -> center-aligned_high_freq_sw1/7(epwmclk)
  Data Type Conversion6/1 -> Goto23/1
  From62/1 -> center-aligned_high_freq_sw1/2(Ts)
  From63/1 -> center-aligned_high_freq_sw1/4(CMPB)
  db3/1 -> center-aligned_high_freq_sw1/5(deadband)
  center-aligned_high_freq_sw1/3(SYNCOUT) -> Goto25/1
  center-aligned_high_freq_sw1/1(PWMA) -> Data Type Conversion6/1
  Data Type Conversion7/1 -> Goto24/1
  [cllcx_ps] -> Product/1
  [md_qa] -> Scope/5
  [timebase_ps] -> Scope/4
  [md_qb] -> Scope/6
  [timebase] -> Scope2/1
  [timebase_ps] -> Scope2/2
  Cast To Double/1 -> Divide/1

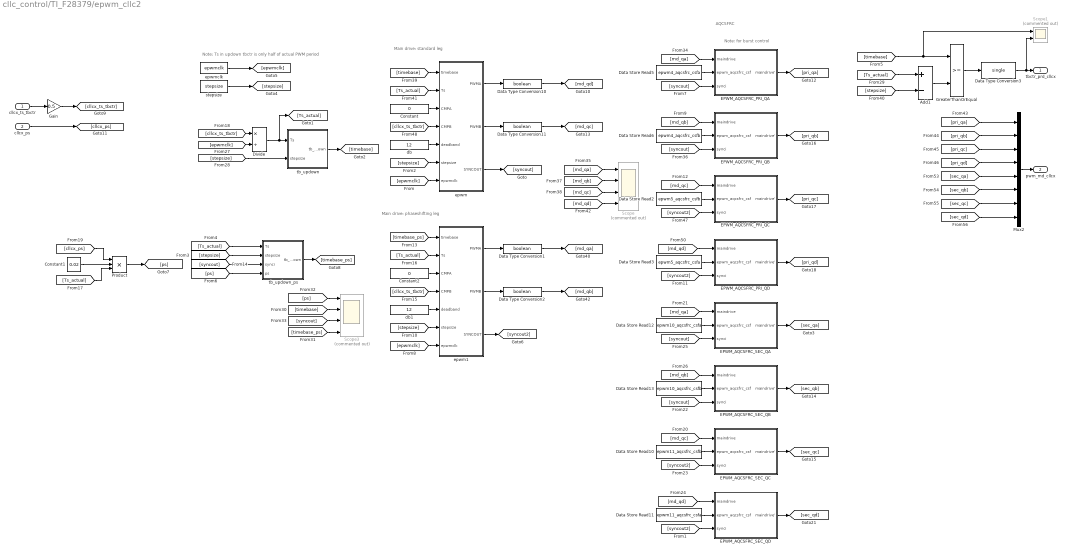
== system cllc_control/TI_F28379/epwm_cllc2 ==
  note: Note: for burst control
  note: AQCSFRC
  note: Main drive: phaseshifting leg
  note: Main drive: standard leg
  note: Note: Ts in updown tbctr is only half of actual PWM period
  cllcx_ts_tbctr : Inport
  cllcx_ps : Inport  Port=2
  Add1 : Sum  Inputs=+-
  Constant : Constant  Value=0
  Constant1 : Constant  Value=0.02
  Constant2 : Constant  Value=0
  Data Store Read10 : DataStoreRead  DataStoreName=epwm11_aqcsfrc_csfb  IndexOptions=Index vector (dialog)  Indices=1  OutputSizes=1
  Data Store Read11 : DataStoreRead  DataStoreName=epwm11_aqcsfrc_csfa  IndexOptions=Index vector (dialog)  Indices=1  OutputSizes=1
  Data Store Read12 : DataStoreRead  DataStoreName=epwm10_aqcsfrc_csfa  IndexOptions=Index vector (dialog)  Indices=1  OutputSizes=1
  Data Store Read13 : DataStoreRead  DataStoreName=epwm10_aqcsfrc_csfb  IndexOptions=Index vector (dialog)  Indices=1  OutputSizes=1
  Data Store Read2 : DataStoreRead  DataStoreName=epwm5_aqcsfrc_csfb  IndexOptions=Index vector (dialog)  Indices=1  OutputSizes=1
  Data Store Read3 : DataStoreRead  DataStoreName=epwm5_aqcsfrc_csfa  IndexOptions=Index vector (dialog)  Indices=1  OutputSizes=1
  Data Store Read5 : DataStoreRead  DataStoreName=epwm4_aqcsfrc_csfa  IndexOptions=Index vector (dialog)  Indices=1  OutputSizes=1
  Data Store Read6 : DataStoreRead  DataStoreName=epwm4_aqcsfrc_csfb  IndexOptions=Index vector (dialog)  Indices=1  OutputSizes=1
  Data Type Conversion{1..2,10..11} (4 alike) : DataTypeConversion  OutDataTypeStr=boolean  SaturateOnIntegerOverflow=off  RndMeth=Floor
  Data Type Conversion3 : DataTypeConversion  OutDataTypeStr=single  SaturateOnIntegerOverflow=off  RndMeth=Floor
  Divide : Product  Inputs=*/
  EPWM_AQCSFRC_PRI_QA : Subsystem  TreatAsAtomicUnit=on
  EPWM_AQCSFRC_PRI_QB : Subsystem  TreatAsAtomicUnit=on
  EPWM_AQCSFRC_PRI_QC : Subsystem  TreatAsAtomicUnit=on
  EPWM_AQCSFRC_PRI_QD : Subsystem  TreatAsAtomicUnit=on
  EPWM_AQCSFRC_SEC_QA : Subsystem  TreatAsAtomicUnit=on
  EPWM_AQCSFRC_SEC_QB : Subsystem  TreatAsAtomicUnit=on
  EPWM_AQCSFRC_SEC_QC : Subsystem  TreatAsAtomicUnit=on
  EPWM_AQCSFRC_SEC_QD : Subsystem  TreatAsAtomicUnit=on
  Gain : Gain  Gain=0.5
  GreaterThanOrEqual : RelationalOperator  OutDataTypeStr=boolean  RndMeth=Simplest  InputSameDT=off
  Mux2 : Mux  Inputs=8
  Product : Product  Inputs=3
  Scope : Scope  Commented=on  NumInputPorts=4
  Scope1 : Scope  Commented=on  NumInputPorts=2
  Scope3 : Scope  Commented=on  NumInputPorts=4
  db : Constant  Value=12
  db1 : Constant  Value=12
  epwm : MATLAB Function  TreatAsAtomicUnit=on
  epwm1 : MATLAB Function  TreatAsAtomicUnit=on
  epwmclk : Constant  Value=epwmclk
  stepsize : Constant  Value=stepsize
  tb_updown : Subsystem
  tb_updown_ps : Subsystem
  tbctr_prd_cllcx : Outport
  pwm_md_cllcx : Outport  Port=2
  wires:
  [syncout] -> EPWM_AQCSFRC_SEC_QA/3(synci)
  [md_qa] -> EPWM_AQCSFRC_SEC_QA/1(maindrive)
  Data Store Read12/1 -> EPWM_AQCSFRC_SEC_QA/2(epwm_aqcsfrc_csf)
  [md_qb] -> EPWM_AQCSFRC_SEC_QB/1(maindrive)
  Data Store Read13/1 -> EPWM_AQCSFRC_SEC_QB/2(epwm_aqcsfrc_csf)
  [syncout] -> EPWM_AQCSFRC_SEC_QB/3(synci)
  [syncout2] -> EPWM_AQCSFRC_SEC_QD/3(synci)
  [syncout2] -> EPWM_AQCSFRC_SEC_QC/3(synci)
  Data Store Read10/1 -> EPWM_AQCSFRC_SEC_QC/2(epwm_aqcsfrc_csf)
  Data Store Read11/1 -> EPWM_AQCSFRC_SEC_QD/2(epwm_aqcsfrc_csf)
  [md_qd] -> EPWM_AQCSFRC_SEC_QD/1(maindrive)
  [md_qc] -> EPWM_AQCSFRC_SEC_QC/1(maindrive)
  EPWM_AQCSFRC_SEC_QA/1(maindrive') -> [sec_qa]
  EPWM_AQCSFRC_SEC_QB/1(maindrive') -> [sec_qb]
  EPWM_AQCSFRC_SEC_QC/1(maindrive') -> [sec_qc]
  EPWM_AQCSFRC_SEC_QD/1(maindrive') -> [sec_qd]
  [sec_qd] -> Mux2/8
  [sec_qc] -> Mux2/7
  [sec_qb] -> Mux2/6
  [sec_qa] -> Mux2/5
  [pri_qa] -> Mux2/1
  [pri_qb] -> Mux2/2
  [pri_qc] -> Mux2/3
  [pri_qd] -> Mux2/4
  EPWM_AQCSFRC_PRI_QD/1(maindrive') -> [pri_qd]
  EPWM_AQCSFRC_PRI_QC/1(maindrive') -> [pri_qc]
  EPWM_AQCSFRC_PRI_QB/1(maindrive') -> [pri_qb]
  EPWM_AQCSFRC_PRI_QA/1(maindrive') -> [pri_qa]
  [md_qc] -> EPWM_AQCSFRC_PRI_QC/1(maindrive)
  [md_qd] -> EPWM_AQCSFRC_PRI_QD/1(maindrive)
  Data Store Read3/1 -> EPWM_AQCSFRC_PRI_QD/2(epwm_aqcsfrc_csf)
  Data Store Read2/1 -> EPWM_AQCSFRC_PRI_QC/2(epwm_aqcsfrc_csf)
  [syncout2] -> EPWM_AQCSFRC_PRI_QC/3(synci)
  [syncout2] -> EPWM_AQCSFRC_PRI_QD/3(synci)
  epwm1/3(SYNCOUT) -> [syncout2]
  [syncout] -> EPWM_AQCSFRC_PRI_QB/3(synci)
  Data Store Read6/1 -> EPWM_AQCSFRC_PRI_QB/2(epwm_aqcsfrc_csf)
  [md_qb] -> EPWM_AQCSFRC_PRI_QB/1(maindrive)
  Data Store Read5/1 -> EPWM_AQCSFRC_PRI_QA/2(epwm_aqcsfrc_csf)
  [md_qd] -> Scope/4
  [md_qc] -> Scope/3
  [md_qb] -> Scope/2
  [md_qa] -> Scope/1
  [md_qa] -> EPWM_AQCSFRC_PRI_QA/1(maindrive)
  [syncout] -> EPWM_AQCSFRC_PRI_QA/3(synci)
  [timebase] -> Scope3/2
  [ps] -> Scope3/1
  [syncout] -> Scope3/3
  [timebase_ps] -> Scope3/4
  Add1/1 -> GreaterThanOrEqual/2
  [Ts_actual] -> Add1/1
  [stepsize] -> Add1/2
  [stepsize] -> tb_updown/2(stepsize)
  [epwmclk] -> Divide/2
  GreaterThanOrEqual/1 -> Data Type Conversion3/1
  Data Type Conversion3/1 -> tbctr_prd_cllcx/1, Scope1/2
  [timebase] -> Scope1/1, GreaterThanOrEqual/1
  [cllcx_ps] -> Product/1
  cllcx_ts_tbctr/1 -> Gain/1
  Constant1/1 -> Product/2
  Product/1 -> [ps]
  [Ts_actual] -> Product/3
  [cllcx_ts_tbctr] -> epwm1/4(CMPB)
  epwm1/2(PWMB) -> Data Type Conversion2/1
  epwm1/1(PWMA) -> Data Type Conversion1/1
  [Ts_actual] -> epwm1/2(Ts)
  Constant2/1 -> epwm1/3(CMPA)
  [timebase_ps] -> epwm1/1(timebase)
  db1/1 -> epwm1/5(deadband)
  [stepsize] -> epwm1/6(stepsize)
  [epwmclk] -> epwm1/7(epwmclk)
  [ps] -> tb_updown_ps/4(ps)
  [syncout] -> tb_updown_ps/3(synci)
  [Ts_actual] -> tb_updown_ps/1(Ts)
  [stepsize] -> tb_updown_ps/2(stepsize)
  tb_updown_ps/1(tb_updown) -> [timebase_ps]
  epwm/3(SYNCOUT) -> [syncout]
  cllcx_ps/1 -> [cllcx_ps]
  [epwmclk] -> epwm/7(epwmclk)
  epwmclk/1 -> [epwmclk]
  [stepsize] -> epwm/6(stepsize)
  db/1 -> epwm/5(deadband)
  [timebase] -> epwm/1(timebase)
  [Ts_actual] -> epwm/2(Ts)
  epwm/1(PWMA) -> Data Type Conversion10/1
  epwm/2(PWMB) -> Data Type Conversion11/1
  stepsize/1 -> [stepsize]
  Divide/1 -> tb_updown/1(Ts), [Ts_actual]
  [cllcx_ts_tbctr] -> Divide/1
  Mux2/1 -> pwm_md_cllcx/1
  tb_updown/1(tb_updown) -> [timebase]
  Constant/1 -> epwm/3(CMPA)
  [cllcx_ts_tbctr] -> epwm/4(CMPB)
  Data Type Conversion10/1 -> [md_qd]
  Data Type Conversion11/1 -> [md_qc]
  Data Type Conversion1/1 -> [md_qa]
  Data Type Conversion2/1 -> [md_qb]
  Gain/1 -> [cllcx_ts_tbctr]

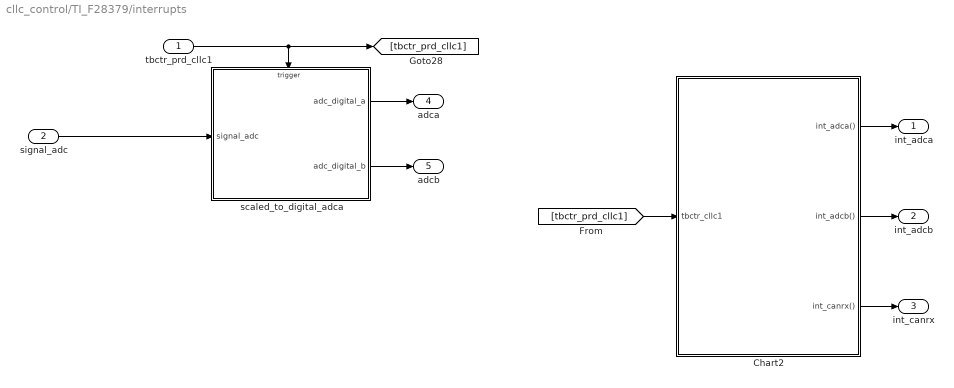
== system cllc_control/TI_F28379/interrupts ==
  tbctr_prd_cllc1 : Inport
  signal_adc : Inport  Port=2
  Chart2 : Stateflow chart  TreatAsAtomicUnit=on
  scaled_to_digital_adca : Subsystem
  int_adca : Outport
  int_adcb : Outport  Port=2
  int_canrx : Outport  Port=3
  adca : Outport  Port=4
  adcb : Outport  Port=5
  wires:
  tbctr_prd_cllc1/1 -> [tbctr_prd_cllc1], scaled_to_digital_adca/Trigger
  scaled_to_digital_adca/1(adc_digital_a) -> adca/1
  signal_adc/1 -> scaled_to_digital_adca/1(signal_adc)
  Chart2/1(int_adca()) -> int_adca/1
  Chart2/2(int_adcb()) -> int_adcb/1
  [tbctr_prd_cllc1] -> Chart2/1(tbctr_cllc1)
  Chart2/3(int_canrx()) -> int_canrx/1
  scaled_to_digital_adca/2(adc_digital_b) -> adcb/1

== system cllc_control/TI_F28379/clb1/pwm_md_trig ==
  Reset : ResetPort  DisableCoverage=on
  Chart : Stateflow chart  TreatAsAtomicUnit=on
  pwm_md_trig : Outport
  wires:
  Chart/1(OUT) -> pwm_md_trig/1

== system cllc_control/TI_F28379/clb2/pwm_md_trig ==
  Reset : ResetPort  DisableCoverage=on
  Chart : Stateflow chart  TreatAsAtomicUnit=on
  pwm_md_trig : Outport
  wires:
  Chart/1(OUT) -> pwm_md_trig/1

== system cllc_control/TI_F28379/clb3/pwm_md_trig ==
  Reset : ResetPort  DisableCoverage=on
  Chart : Stateflow chart  TreatAsAtomicUnit=on
  pwm_md_trig : Outport
  wires:
  Chart/1(OUT) -> pwm_md_trig/1

== system cllc_control/TI_F28379/clb4/pwm_md_trig ==
  Reset : ResetPort  DisableCoverage=on
  Chart : Stateflow chart  TreatAsAtomicUnit=on
  pwm_md_trig : Outport
  wires:
  Chart/1(OUT) -> pwm_md_trig/1

== system cllc_control/TI_F28379/epwm_cllc1/EPWM_AQCSFRC_PRI_QA ==
  maindrive : Inport
  epwm_aqcsfrc_csf : Inport  Port=2
  synci : Inport  Port=3
  Cast To Boolean : DataTypeConversion  OutDataTypeStr=boolean  SaturateOnIntegerOverflow=off  RndMeth=Floor
  NOT4 : Logic  Operator=NOT  IconShape=distinctive  AllPortsSameDT=off  OutDataTypeStr=boolean
  Product2 : Product
  Sample and Hold1 : spsSampleandHoldLib/Sample and Hold  ic=0  Ts=0
      settings: SourceProductBaseCode=PS
  maindrive' : Outport  PortDimensions=[1 1]
  wires:
  epwm_aqcsfrc_csf/1 -> NOT4/1
  maindrive/1 -> Product2/1
  NOT4/1 -> Sample and Hold1/1
  synci/1 -> Sample and Hold1/2
  Product2/1 -> Cast To Boolean/1
  Sample and Hold1/1 -> Product2/2
  Cast To Boolean/1 -> maindrive'/1

== system cllc_control/TI_F28379/epwm_cllc1/EPWM_AQCSFRC_PRI_QB ==
  maindrive : Inport
  epwm_aqcsfrc_csf : Inport  Port=2
  synci : Inport  Port=3
  Cast To Boolean : DataTypeConversion  OutDataTypeStr=boolean  SaturateOnIntegerOverflow=off  RndMeth=Floor
  NOT4 : Logic  Operator=NOT  IconShape=distinctive  AllPortsSameDT=off  OutDataTypeStr=boolean
  Product2 : Product
  Sample and Hold1 : spsSampleandHoldLib/Sample and Hold  ic=0  Ts=0
      settings: SourceProductBaseCode=PS
  maindrive' : Outport  PortDimensions=[1 1]
  wires:
  Sample and Hold1/1 -> Product2/2
  Product2/1 -> Cast To Boolean/1
  synci/1 -> Sample and Hold1/2
  NOT4/1 -> Sample and Hold1/1
  maindrive/1 -> Product2/1
  epwm_aqcsfrc_csf/1 -> NOT4/1
  Cast To Boolean/1 -> maindrive'/1

== system cllc_control/TI_F28379/epwm_cllc1/EPWM_AQCSFRC_PRI_QC ==
  maindrive : Inport
  epwm_aqcsfrc_csf : Inport  Port=2
  synci : Inport  Port=3
  Cast To Boolean : DataTypeConversion  OutDataTypeStr=boolean  SaturateOnIntegerOverflow=off  RndMeth=Floor
  NOT4 : Logic  Operator=NOT  IconShape=distinctive  AllPortsSameDT=off  OutDataTypeStr=boolean
  Product2 : Product
  Sample and Hold1 : spsSampleandHoldLib/Sample and Hold  ic=0  Ts=0
      settings: SourceProductBaseCode=PS
  maindrive' : Outport  PortDimensions=[1 1]
  wires:
  Sample and Hold1/1 -> Product2/2
  Product2/1 -> Cast To Boolean/1
  synci/1 -> Sample and Hold1/2
  NOT4/1 -> Sample and Hold1/1
  maindrive/1 -> Product2/1
  epwm_aqcsfrc_csf/1 -> NOT4/1
  Cast To Boolean/1 -> maindrive'/1

== system cllc_control/TI_F28379/epwm_cllc1/EPWM_AQCSFRC_PRI_QD ==
  maindrive : Inport
  epwm_aqcsfrc_csf : Inport  Port=2
  synci : Inport  Port=3
  Cast To Boolean : DataTypeConversion  OutDataTypeStr=boolean  SaturateOnIntegerOverflow=off  RndMeth=Floor
  NOT4 : Logic  Operator=NOT  IconShape=distinctive  AllPortsSameDT=off  OutDataTypeStr=boolean
  Product2 : Product
  Sample and Hold1 : spsSampleandHoldLib/Sample and Hold  ic=0  Ts=0
      settings: SourceProductBaseCode=PS
  maindrive' : Outport  PortDimensions=[1 1]
  wires:
  epwm_aqcsfrc_csf/1 -> NOT4/1
  maindrive/1 -> Product2/1
  NOT4/1 -> Sample and Hold1/1
  synci/1 -> Sample and Hold1/2
  Product2/1 -> Cast To Boolean/1
  Sample and Hold1/1 -> Product2/2
  Cast To Boolean/1 -> maindrive'/1

== system cllc_control/TI_F28379/epwm_cllc1/EPWM_AQCSFRC_SEC_QA ==
  maindrive : Inport
  epwm_aqcsfrc_csf : Inport  Port=2
  synci : Inport  Port=3
  Cast To Boolean : DataTypeConversion  OutDataTypeStr=boolean  SaturateOnIntegerOverflow=off  RndMeth=Floor
  NOT4 : Logic  Operator=NOT  IconShape=distinctive  AllPortsSameDT=off  OutDataTypeStr=boolean
  Product2 : Product
  Sample and Hold1 : spsSampleandHoldLib/Sample and Hold  ic=0  Ts=0
      settings: SourceProductBaseCode=PS
  maindrive' : Outport  PortDimensions=[1 1]
  wires:
  Cast To Boolean/1 -> maindrive'/1
  Sample and Hold1/1 -> Product2/2
  Product2/1 -> Cast To Boolean/1
  synci/1 -> Sample and Hold1/2
  NOT4/1 -> Sample and Hold1/1
  maindrive/1 -> Product2/1
  epwm_aqcsfrc_csf/1 -> NOT4/1

== system cllc_control/TI_F28379/epwm_cllc1/EPWM_AQCSFRC_SEC_QB ==
  maindrive : Inport
  epwm_aqcsfrc_csf : Inport  Port=2
  synci : Inport  Port=3
  Cast To Boolean : DataTypeConversion  OutDataTypeStr=boolean  SaturateOnIntegerOverflow=off  RndMeth=Floor
  NOT4 : Logic  Operator=NOT  IconShape=distinctive  AllPortsSameDT=off  OutDataTypeStr=boolean
  Product2 : Product
  Sample and Hold1 : spsSampleandHoldLib/Sample and Hold  ic=0  Ts=0
      settings: SourceProductBaseCode=PS
  maindrive' : Outport  PortDimensions=[1 1]
  wires:
  Cast To Boolean/1 -> maindrive'/1
  epwm_aqcsfrc_csf/1 -> NOT4/1
  maindrive/1 -> Product2/1
  NOT4/1 -> Sample and Hold1/1
  synci/1 -> Sample and Hold1/2
  Product2/1 -> Cast To Boolean/1
  Sample and Hold1/1 -> Product2/2

== system cllc_control/TI_F28379/epwm_cllc1/EPWM_AQCSFRC_SEC_QC ==
  maindrive : Inport
  epwm_aqcsfrc_csf : Inport  Port=2
  synci : Inport  Port=3
  Cast To Boolean : DataTypeConversion  OutDataTypeStr=boolean  SaturateOnIntegerOverflow=off  RndMeth=Floor
  NOT4 : Logic  Operator=NOT  IconShape=distinctive  AllPortsSameDT=off  OutDataTypeStr=boolean
  Product2 : Product
  Sample and Hold1 : spsSampleandHoldLib/Sample and Hold  ic=0  Ts=0
      settings: SourceProductBaseCode=PS
  maindrive' : Outport  PortDimensions=[1 1]
  wires:
  Cast To Boolean/1 -> maindrive'/1
  epwm_aqcsfrc_csf/1 -> NOT4/1
  maindrive/1 -> Product2/1
  NOT4/1 -> Sample and Hold1/1
  synci/1 -> Sample and Hold1/2
  Product2/1 -> Cast To Boolean/1
  Sample and Hold1/1 -> Product2/2
